simulink subsystem "ct_control_ref_subsys"  (R2022b)
settings: Solver=VariableStepAuto  StartTime=0.0  StopTime=10.0  RelTol=1e-3
undefined symbols (not defined in the file): ctrl_param, param_robot
settings Model: Creator=emu  LastModifiedBy=emu

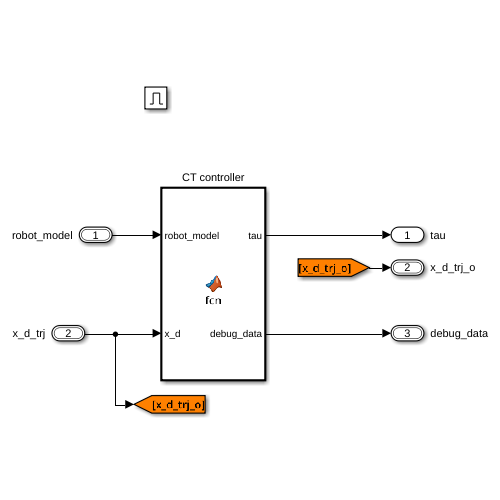
[thumbnail: Simulink's stored preview of the top-level diagram]
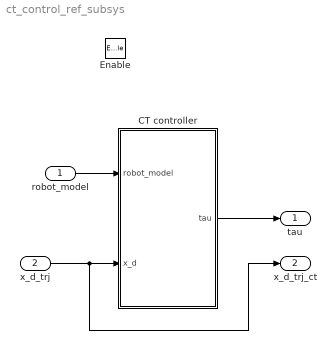
== system ct_control_ref_subsys ==
  robot_model : Inport  OutDataTypeStr=Bus: robot_model
  x_d_trj : Inport  Port=2  OutDataTypeStr=Bus: x_d
  Enable : EnablePort
  CT controller : MATLAB Function  TreatAsAtomicUnit=on
  tau : Outport
  x_d_trj_ct : Outport  Port=2  OutDataTypeStr=Bus: x_d
  wires:
  x_d_trj/1 -> CT controller/2(x_d), x_d_trj_ct/1
  CT controller/1(tau) -> tau/1
  robot_model/1 -> CT controller/1(robot_model)

== matlab function ct_control_ref_subsys/CT controller ==
  settings: updateMethod=DISCRETE  sampleTime=param_global.Ta
  data: tau output; robot_model input Bus: robot_model; x_d input Bus: x_d; ctrl_param parameter; param_robot parameter
function tau  = fcn(robot_model, x_d, ctrl_param, param_robot)

% Parameters
%q = robot_model.q;      % generalized coordinates
q_p = robot_model.q_p;  % time derivative of generalized coordinates

M = robot_model.M;      % inertia matrix
%C = robot_model.C;      % coriolis matrix
%g = robot_model.g;      % gravitational forces
%C_rnea = C*q_p + g;
C_rnea = robot_model.C_rnea; % C_rnea(q, q_p) = C(q, q_p)q_p + g(q) = n(q, q_p)

J = robot_model.J;      % geometric jacobian to end-effector
J_p = robot_model.J_p;  % time derivative of geometric jacobian to end-effector

H = robot_model.H;

n = param_robot.n_red;
n_indices = param_robot.n_indices;

yt_indices = param_robot.yt_indices;
yr_indices = param_robot.yr_indices;
y_indices =  [yt_indices 3+yr_indices];

m = numel(yt_indices) + numel(yr_indices);

M_red = M(n_indices, n_indices);
C_rnea_red = C_rnea(n_indices);

J_red = J(y_indices, n_indices);
J_p_red = J_p(y_indices, :);

% Control parameters
Kp1 = ctrl_param.ct.Kp1(y_indices, y_indices);
Kd1 = ctrl_param.ct.Kd1(y_indices, y_indices);

% Current Pose of Endeffector
x_p = J*q_p;

p = H(yt_indices,4);
R = H(1:3,1:3);
p_p  = x_p(yt_indices);
omega_e = x_p(3+yr_indices); % Drehwinkelgeschwindigkeit des Endeffektors

% Desired Trajectory
p_d    = x_d.p_d(yt_indices);
p_d_p  = x_d.p_d_p(yt_indices);
p_d_pp = x_d.p_d_pp(yt_indices);

R_d = x_d.R_d;
omega_d = x_d.omega_d(yr_indices);
omega_d_p = x_d.omega_d_p(yr_indices);

% Errors
RR = R*R_d';
q_err_tmp   = rotm2quat_v4(RR);
q_err = q_err_tmp(1+yr_indices);

x_err   = [p-p_d;      q_err];   % Error as quaternion
x_err_p = [p_p-p_d_p;  omega_e-omega_d];
x_d_pp  = [p_d_pp;     omega_d_p];


% CT control law
%% Cartesian Endeffector Pose

sing_method = ctrl_param.regularization.mode;

if(sing_method == 0)
    v = J_red\(x_d_pp - Kd1*x_err_p - Kp1*x_err - J_p_red*q_p);
elseif(sing_method == 1) % add +k*E
    k = ctrl_param.regularization.k;
    J_pinv = (J_red'*J_red + k*eye(n))\J_red';
    v = J_pinv * (x_d_pp - Kd1*x_err_p - Kp1*x_err - J_p_red*q_p);
elseif(sing_method == 2) % add +lambda*E
    W_bar_N = ctrl_param.regularization.W_bar_N(n_indices);
    W_E = ctrl_param.regularization.W_E(y_indices, y_indices);

    e = x_err;
    E_k = 1/2 * e' * W_E * e;
    W_N = eye(n)*E_k + W_bar_N;

    [~, S, V] = svd(sqrt(W_E)*J_red);

    S_nonzero = diag(diag(S)); % get only nonzero sing values

    H_k = V*(S_nonzero^2)*V' + W_N;
    J_pinv = H_k\J_red';
    v = J_pinv * (x_d_pp - Kd1*x_err_p - Kp1*x_err - J_p_red*q_p);
    %v = H_k \ J_red' * (x_d_pp - Kd1*x_err_p - Kp1*x_err - J_p*q_p);
elseif(sing_method == 3) % remove small singular values
    % Perform SVD
    [U, S, V] = svd(J_red);
    
    % Set a threshold for small singular values
    epsilon = ctrl_param.regularization.eps; % Adjust epsilon as needed
    
    % Threshold small singular values in S
    S_new = diag(max(diag(S), epsilon));  % Creates a diagonal matrix with thresholded values
    S(1:n, 1:n) = S_new;
    
    % Reconstruct the matrix with modified singular values
    J_new = U * S * V';
    J_pinv = pinv(J_new);
    v = J_pinv * (x_d_pp - Kd1*x_err_p - Kp1*x_err - J_p_red*q_p);
elseif(sing_method == 4) % collinearity   
    if(rank(J_red, 1e-1) < m)
        J_tilde = J_red./vecnorm(J_red);
        JJ_colin = J_tilde'*J_tilde;
        [i,j] = find(abs(tril(JJ_colin) - eye(n)) > ctrl_param.regularization.eps_collinear);

        J_red(:, j) = 0;
        
        J_pinv = pinv(J_red);
        
        v = J_pinv * (x_d_pp - Kd1*x_err_p - Kp1*x_err - J_p_red*q_p);% - D_n * q_p_nullspace - K_n * (q_nullspace - q_d_nullspace);
        v(j) = 0;
    else
        v = J_red \ (x_d_pp - Kd1*x_err_p - Kp1*x_err - J_p_red*q_p);% - D_n * q_p_nullspace - K_n * (q_nullspace - q_d_nullspace);
    end
else%if(sing_method == 5) % nach Steinboeck Optreg
    J_scale = 1./vecnorm(J_red);
    J_tilde = J_red.*J_scale;
    JJ_colin = J_tilde'*J_tilde;
    %[V, D] = eig(JJ_colin);

    [U, D, V] = svd(JJ_colin);

    V_new = real(V(:, real(diag(D)) > ctrl_param.regularization.lambda_min));

    T_bar = J_scale' .* V_new;

    J_new = J_red*T_bar;

    v = T_bar * ( J_new \ (x_d_pp - Kd1*x_err_p - Kp1*x_err - J_p_red*q_p) );
end

tau = M_red*v + C_rnea_red;
%if(max(abs(tau)) > 200)
%    disp('no');
%end
